simulink model "mCoolantDemuxMux"  (R2021b)
settings: Solver=VariableStepAuto  StartTime=0.0  StopTime=10.0  RelTol=1e-3
libraries: mcadROM_lib x4, simulink x4
settings Model: Creator=agonzale  LastModifiedBy=agonzale

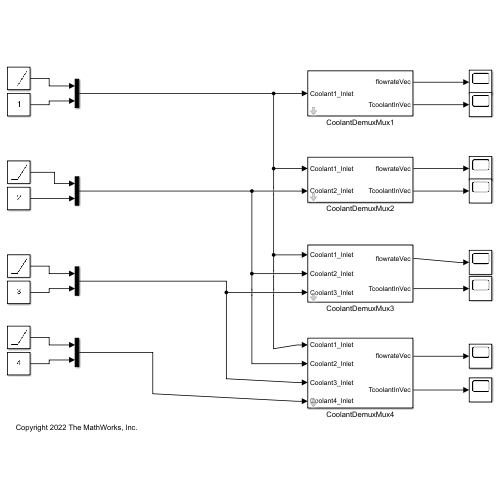
[thumbnail: Simulink's stored preview of the top-level diagram]
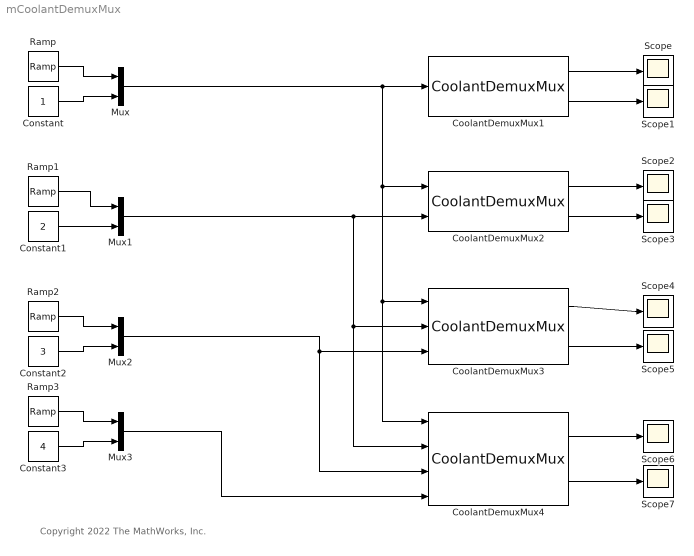
== system mCoolantDemuxMux ==
  note: Copyright 2022 The MathWorks, Inc.
  Constant : Constant
  Constant1 : Constant  Value=2
  Constant2 : Constant  Value=3
  Constant3 : Constant  Value=4
  CoolantDemuxMux1 : mcadROM_lib/CoolantDemuxMux  numCoolSys=1
  CoolantDemuxMux2 : mcadROM_lib/CoolantDemuxMux  numCoolSys=2
  CoolantDemuxMux3 : mcadROM_lib/CoolantDemuxMux  numCoolSys=3
  CoolantDemuxMux4 : mcadROM_lib/CoolantDemuxMux  numCoolSys=4
  Mux{,1..3} (4 alike) : Mux  Inputs=2
  Ramp : simulink/Sources/Ramp  slope=1  start=0  InitialOutput=0
  Ramp1 : simulink/Sources/Ramp  slope=2  start=0  InitialOutput=0
  Ramp2 : simulink/Sources/Ramp  slope=3  start=0  InitialOutput=0
  Ramp3 : simulink/Sources/Ramp  slope=4  start=0  InitialOutput=0
  Scope{,1..7} (8 alike) : Scope
  wires:
  Ramp/1 -> Mux/1
  Constant/1 -> Mux/2
  CoolantDemuxMux1/2 -> Scope1/1
  CoolantDemuxMux1/1 -> Scope/1
  CoolantDemuxMux2/2 -> Scope3/1
  CoolantDemuxMux2/1 -> Scope2/1
  Constant1/1 -> Mux1/2
  Ramp1/1 -> Mux1/1
  Constant2/1 -> Mux2/2
  Ramp2/1 -> Mux2/1
  Constant3/1 -> Mux3/2
  Ramp3/1 -> Mux3/1
  Mux/1 -> CoolantDemuxMux2/1, CoolantDemuxMux4/1, CoolantDemuxMux3/1, CoolantDemuxMux1/1
  Mux1/1 -> CoolantDemuxMux4/2, CoolantDemuxMux3/2, CoolantDemuxMux2/2
  Mux2/1 -> CoolantDemuxMux3/3, CoolantDemuxMux4/3
  Mux3/1 -> CoolantDemuxMux4/4
  CoolantDemuxMux3/2 -> Scope5/1
  CoolantDemuxMux3/1 -> Scope4/1
  CoolantDemuxMux4/2 -> Scope7/1
  CoolantDemuxMux4/1 -> Scope6/1
